simulink model "SalientPolePMSM"  (R2020b)
settings: Solver=VariableStepAuto  StartTime=0  StopTime=1  MaxStep=1e-4  RelTol=1e-4
values from neighbouring files (symbols this model uses):
  Bgain = 1    [DataSalientPolePMSM-DESKTOP-IINSHMA.m]    (also in DataSalientPolePMSM.m)
  Gcc_1ord = 1/(s/bandwidth(Gcc) + 1)    [DataSalientPolePMSM-DESKTOP-IINSHMA.m]    (also in DataSalientPolePMSM.m)
  lamdVec = mot.Ld*idVec+mot.lammg    [DataSalientPolePMSM-DESKTOP-IINSHMA.m]    (also in DataSalientPolePMSM.m)
  lamqVec = mot.Lq*iqVec    [DataSalientPolePMSM-DESKTOP-IINSHMA.m]    (also in DataSalientPolePMSM.m)
  TAB0_abc = Tabc_AB0^-1    [DataSalientPolePMSM-DESKTOP-IINSHMA.m]    (also in DataSalientPolePMSM.m)
  Tabc_AB0 = 2/3.*[     1       -1/2       -1/2 ... (first row only)    [DataSalientPolePMSM-DESKTOP-IINSHMA.m]    (also in DataSalientPolePMSM.m)
  Talphabeta_abc = Tabc_alphabeta^(-1)    [DataSalientPolePMSM-DESKTOP-IINSHMA.m]    (also in DataSalientPolePMSM.m)
undefined symbols (not defined in the file or in its folder): DiscIntNeverNeededParam, dqpll, inv, kid, kpd, magnitude, meas, mot, Obs, PI, stconv
libraries: simulink x53, pid_lib x3, powerlib x2, eeBldcCommutationLogic x1, electricdrivelib x1
(part 2 of 7)

== system SalientPolePMSM/DT SENSORLESS ALGORITHM DQ ==
  note: tangent PLL
  iabc1 : Inport
  udq_est : Inport  Port=2
  udq : Inport  Port=3
  In3 : Inport  Port=4
  thme1 : Inport  Port=5
  wme : Inport  Port=6
  Clarke + Park 5 : Subsystem
      settings: PortSchema="{\"entries\":[{\"content\":{\"sides\":[{\"content\":{\"connectorIds\":[\"In1\"]},\"type\":\"ConnectorPlacement.EquallySpacedRectSide\",\"uuid\":\"e456cd5a-7662-4e0b-a6c7-27ed01a0cde8\"},{\"content\":{\"connectorIds\":[\"Out1\"],\"side\":\"RIGHT\"},\"type\":\"ConnectorPlacement.EquallySpacedRectSide\",\"uuid\":\"028e266b-db3d-4fa0-9acb-55f4e679375c\"},{\"content\":{\"connectorIds\":[],\"side\":\"TOP\"},\"type\":\"ConnectorPlacement.EquallySpacedRectSide\",\"uuid\":\"fc8407b0-ab5c-4984-8f89-848ec890a8d5\"},{\"content\":{\"connectorIds\":[\"In2\"],\"side\":\"BOTTOM\"},\"type\":\"ConnectorPlacement.EquallySpacedRectSide\",\"uuid\":\"5b71beec-2170-4cb0-81b8-756f92b052d7\"},{\"content\":{\"connectorIds\":[],\"side\":\"HIDDEN\"},\"type\":\"ConnectorPlacement.EquallySpacedRectSide\",\"uuid\":\"110705d2-59f3-422e-b935-78b651f69ef1\"}]},\"type\":\"ConnectorPlacement.EquallySpacedConnector\",\"uuid\":\"4a76e66d-c848-4e9c-8e50-4d720647e920\"}],\"packageUris\":[\"http://schema.mathworks.com/mf0/Connector/R2020b\"],\"version\":\"1.0\"}"
  Classic PLL1 : Subsystem
  DECOUPLING : Subsystem
      settings: PortSchema="{\"entries\":[{\"content\":{\"sides\":[{\"content\":{\"connectorIds\":[\"In1\",\"In2\"]},\"type\":\"ConnectorPlacement.EquallySpacedRectSide\",\"uuid\":\"11caacf5-0bb5-4a8d-b3e9-7b1e88488e40\"},{\"content\":{\"connectorIds\":[\"Out1\",\"Out2\"],\"side\":\"RIGHT\"},\"type\":\"ConnectorPlacement.EquallySpacedRectSide\",\"uuid\":\"6263df69-80cd-4b04-a89b-dfca9161a93e\"},{\"content\":{\"connectorIds\":[],\"side\":\"TOP\"},\"type\":\"ConnectorPlacement.EquallySpacedRectSide\",\"uuid\":\"898c91db-8461-4171-8db9-87a99b66ce40\"},{\"content\":{\"connectorIds\":[\"In3\"],\"side\":\"BOTTOM\"},\"type\":\"ConnectorPlacement.EquallySpacedRectSide\",\"uuid\":\"185c1e28-6dbc-44e9-9bab-ce833de258e7\"},{\"content\":{\"connectorIds\":[],\"side\":\"HIDDEN\"},\"type\":\"ConnectorPlacement.EquallySpacedRectSide\",\"uuid\":\"0f2378b2-18e5-4bfa-bdaa-e448fe90a90d\"}]},\"type\":\"ConnectorPlacement.EquallySpacedConnector\",\"uuid\":\"5ac053f8-067e-460f-b603-fa451a6d3395\"}],\"packageUris\":[\"http://schema.mathworks.com/mf0/Connector/R2020b\"],\"version\":\"1.0\"}"
  Discrete Filter1 : DiscreteFilter  Numerator=[Obs.lpf.alpha*10]  Denominator=[1 ((Obs.lpf.alpha*10)-1)]  SampleTime=Obs.Ts
  Discrete Filter2 : DiscreteFilter  Commented=on  Numerator=[Obs.lpf.alpha]  Denominator=[1 (Obs.lpf.alpha-1)]  SampleTime=100e-6
  Discrete State-Space3 : DiscreteStateSpace  A=Obs.F1  B=Obs.G1  C=Obs.H1  D=Obs.D1  SampleTime=100e-6
  Discrete State-Space4 : DiscreteStateSpace  A=Obs.F1  B=Obs.G1  C=Obs.H1  D=Obs.D1  SampleTime=100e-6
  Discrete-Time Integrator : DiscreteIntegrator  gainval=1  SampleTime=100e-6  ICPrevOutput=DiscIntNeverNeededParam  ICPrevScaledInput=DiscIntNeverNeededParam
  Integrator : Integrator
  MATLAB Function1 : MATLAB Function  TreatAsAtomicUnit=on
  Normalized and improved PLL3 : Subsystem
  PII : Subsystem
      settings: PortSchema="{\"entries\":[{\"content\":{\"sides\":[{\"content\":{\"connectorIds\":[\"In1\"]},\"type\":\"ConnectorPlacement.EquallySpacedRectSide\",\"uuid\":\"b00016c6-1c57-43c7-9cfb-2a554e77d147\"},{\"content\":{\"connectorIds\":[\"Out1\"],\"side\":\"RIGHT\"},\"type\":\"ConnectorPlacement.EquallySpacedRectSide\",\"uuid\":\"2a623ad0-8b44-45a2-8fa5-d5134e76836f\"},{\"content\":{\"connectorIds\":[\"In2\"],\"side\":\"TOP\"},\"type\":\"ConnectorPlacement.EquallySpacedRectSide\",\"uuid\":\"30b77249-c9f6-4999-a309-d04d29204cea\"},{\"content\":{\"connectorIds\":[],\"side\":\"HIDDEN\"},\"type\":\"ConnectorPlacement.EquallySpacedRectSide\",\"uuid\":\"35f0e0cd-3c1e-4861-ab0d-8c8ad5904a85\"}]},\"type\":\"ConnectorPlacement.EquallySpacedConnector\",\"uuid\":\"0e7458ac-b887-4f57-92cf-b77cd1ee8214\"}],\"packageUris\":[\"http://schema.mathworks.com/mf0/Connector/R2020b\"],\"version\":\"1.0\"}"
  Rate Transition{,13..15} (4 alike) : RateTransition
  Rev_Park + Rev_Clarke1 : Subsystem
      settings: PortSchema="{\"entries\":[{\"content\":{\"sides\":[{\"content\":{\"connectorIds\":[\"In1\"]},\"type\":\"ConnectorPlacement.EquallySpacedRectSide\",\"uuid\":\"2aae3f04-c402-455e-9a5d-4c573bec95dc\"},{\"content\":{\"connectorIds\":[\"Out1\"],\"side\":\"RIGHT\"},\"type\":\"ConnectorPlacement.EquallySpacedRectSide\",\"uuid\":\"f1532c60-2267-456b-9c2f-34e60e60798d\"},{\"content\":{\"connectorIds\":[],\"side\":\"TOP\"},\"type\":\"ConnectorPlacement.EquallySpacedRectSide\",\"uuid\":\"04e1a6cc-513a-47f7-a63d-759add73a2e3\"},{\"content\":{\"connectorIds\":[\"In2\"],\"side\":\"BOTTOM\"},\"type\":\"ConnectorPlacement.EquallySpacedRectSide\",\"uuid\":\"e4fadd8d-bc98-4107-9436-b30fd69f2e4f\"},{\"content\":{\"connectorIds\":[],\"side\":\"HIDDEN\"},\"type\":\"ConnectorPlacement.EquallySpacedRectSide\",\"uuid\":\"086bd472-9627-4f82-bc83-4764e9943a88\"}]},\"type\":\"ConnectorPlacement.EquallySpacedConnector\",\"uuid\":\"0de85400-6c41-4ce8-8482-fdca09eb4650\"}],\"packageUris\":[\"http://schema.mathworks.com/mf0/Connector/R2020b\"],\"version\":\"1.0\"}"
  Scope : Scope  NumInputPorts=5
  Scope1 : Scope  NumInputPorts=3
  Scope2 : Scope
  Scope3 : Scope  NumInputPorts=3
  atan : MATLAB Function  TreatAsAtomicUnit=on
  thme_est : Outport
  wme_est : Outport  Port=2
  wires:
  Rate Transition14/1 -> Rev_Park + Rev_Clarke1/1(Iabc)
  Rate Transition15/1 -> Clarke + Park 5/1(abc)
  Rev_Park + Rev_Clarke1/1(dq) -> Scope2/1, DECOUPLING/1(idq_est)
  iabc1/1 -> Rate Transition14/1
  Rate Transition13/1 -> wme_est/1
  Discrete State-Space4/1 -> Classic PLL1/1(e_d), atan/1(ed), Scope/3
  Discrete State-Space3/1 -> Classic PLL1/2(e_q), atan/2(eq), Scope/4
  atan/1(thme) -> Scope3/3, PII/1(theta(k+1))
  DECOUPLING/1(ud' id) -> Scope/2, Discrete State-Space4/1
  DECOUPLING/2(uq' iq) -> Scope/1, Discrete State-Space3/1
  In3/1 -> Rate Transition15/1
  [THME_EST] -> Clarke + Park 5/2(thme)
  thme1/1 -> Scope3/1
  Discrete Filter1/1 -> Rate Transition13/1, DECOUPLING/3(wme_est)
  Rate Transition/1 -> thme_est/1
  Discrete-Time Integrator/1 -> Scope3/2, [THME_EST], Rate Transition/1
  PII/1(w_est) -> Discrete Filter1/1, Discrete-Time Integrator/1, MATLAB Function1/1(u)
  [THME_EST] -> Rev_Park + Rev_Clarke1/2(thme1)
  Clarke + Park 5/1(dq) -> DECOUPLING/2(udq_est)

== system SalientPolePMSM/Decoupling ==
  note: OUTPUT:
  note: INPUTS:
  udq* : Inport
  idq : Inport  Port=2
  wme : Inport  Port=3
  Demux : Demux  Outputs=2
  Demux1 : Demux  Outputs=2
  Demux2 : Demux  Outputs=2
  Gain : Gain  Gain=PI.cur.Ld
  Gain1 : Gain  Gain=PI.cur.Lq
  Gain2 : Gain  Gain=PI.cur.lammg
  Mux : Mux  Inputs=2
  Product : Product
  Product1 : Product
  Scope : Scope
  Scope1 : Scope
  Subtract : Sum  Inputs=-+
  Subtract1 : Sum  Inputs=+++
  Terminator1 : Terminator
  Terminator4 : Terminator
  idq1 : InportShadow  Port=2
  wme1 : InportShadow  Port=3
  udq** : Outport
  wires:
  Demux2/1 -> Product/2  "id"
  idq/1 -> Demux2/1
  Product/1 -> Subtract1/3  "wme*id*Ld"
  Subtract/1 -> Scope/1, Mux/1
  Demux/2 -> Subtract1/1
  Demux2/2 -> Terminator1/1
  Demux/1 -> Subtract/2
  wme/1 -> Gain/1, Gain2/1
  Subtract1/1 -> Scope1/1, Mux/2
  Gain2/1 -> Subtract1/2  "wme*lammg"
  Gain/1 -> Product/1
  Mux/1 -> udq**/1
  udq*/1 -> Demux/1
  Demux1/2 -> Product1/1  "iq"
  idq1/1 -> Demux1/1
  Demux1/1 -> Terminator4/1
  Gain1/1 -> Product1/2
  wme1/1 -> Gain1/1
  Product1/1 -> Subtract/1  "wme*iq*Lq"

== system SalientPolePMSM/Discrete SS ALGORITHM ==
  iabc : Inport
  uabc : Inport  Port=2
  ON_approx : Inport  Port=3
  ADD_integrator : Inport  Port=4
  DECOUPLING : Subsystem
      settings: PortSchema="{\"entries\":[{\"content\":{\"sides\":[{\"content\":{\"connectorIds\":[\"In1\",\"In2\"]},\"type\":\"ConnectorPlacement.EquallySpacedRectSide\",\"uuid\":\"11caacf5-0bb5-4a8d-b3e9-7b1e88488e40\"},{\"content\":{\"connectorIds\":[\"Out1\",\"Out2\"],\"side\":\"RIGHT\"},\"type\":\"ConnectorPlacement.EquallySpacedRectSide\",\"uuid\":\"6263df69-80cd-4b04-a89b-dfca9161a93e\"},{\"content\":{\"connectorIds\":[],\"side\":\"TOP\"},\"type\":\"ConnectorPlacement.EquallySpacedRectSide\",\"uuid\":\"898c91db-8461-4171-8db9-87a99b66ce40\"},{\"content\":{\"connectorIds\":[\"In3\"],\"side\":\"BOTTOM\"},\"type\":\"ConnectorPlacement.EquallySpacedRectSide\",\"uuid\":\"185c1e28-6dbc-44e9-9bab-ce833de258e7\"},{\"content\":{\"connectorIds\":[],\"side\":\"HIDDEN\"},\"type\":\"ConnectorPlacement.EquallySpacedRectSide\",\"uuid\":\"0f2378b2-18e5-4bfa-bdaa-e448fe90a90d\"}]},\"type\":\"ConnectorPlacement.EquallySpacedConnector\",\"uuid\":\"5ac053f8-067e-460f-b603-fa451a6d3395\"}],\"packageUris\":[\"http://schema.mathworks.com/mf0/Connector/R2020b\"],\"version\":\"1.0\"}"
  Demux : Demux  Outputs=2
  Discrete Filter2 : DiscreteFilter  Numerator=[dqpll.lpf.alpha]  Denominator=[1 (dqpll.lpf.alpha-1)]
  Discrete State-Space1 : DiscreteStateSpace  A=dqpll.est.F1  B=dqpll.est.G1  C=dqpll.est.H1  D=dqpll.est.D1  SampleTime=dqpll.Ts
  Discrete State-Space2 : DiscreteStateSpace  A=dqpll.est.F1  B=dqpll.est.G1  C=dqpll.est.H1  D=dqpll.est.D1  SampleTime=dqpll.Ts
  Discrete-Time Integrator1 : DiscreteIntegrator  gainval=1  SampleTime=dqpll.Ts  ICPrevOutput=DiscIntNeverNeededParam  ICPrevScaledInput=DiscIntNeverNeededParam
  MATLAB Function3 : MATLAB Function  TreatAsAtomicUnit=on
  PI : Subsystem
  PII : Subsystem
  Rate Transition{,1..5} (6 alike) : RateTransition
  Scope : Scope  NumInputPorts=2
  Scope1 : Scope  NumInputPorts=2
  Subsystem5 : Subsystem
      settings: PortSchema="{\"entries\":[{\"content\":{\"sides\":[{\"content\":{\"connectorIds\":[\"In1\"]},\"type\":\"ConnectorPlacement.EquallySpacedRectSide\",\"uuid\":\"4ed90ab9-1fa1-426e-9a51-633f86eaed93\"},{\"content\":{\"connectorIds\":[\"Out1\"],\"side\":\"RIGHT\"},\"type\":\"ConnectorPlacement.EquallySpacedRectSide\",\"uuid\":\"a783641a-eefd-4804-96bc-e093b09f1b23\"},{\"content\":{\"connectorIds\":[\"In2\"],\"side\":\"TOP\"},\"type\":\"ConnectorPlacement.EquallySpacedRectSide\",\"uuid\":\"b71fad55-6d7c-4fa9-b8c9-7c2d781b5980\"},{\"content\":{\"connectorIds\":[],\"side\":\"BOTTOM\"},\"type\":\"ConnectorPlacement.EquallySpacedRectSide\",\"uuid\":\"0ef0ee48-37c5-4f1f-a4a0-75388778f62a\"},{\"content\":{\"connectorIds\":[],\"side\":\"HIDDEN\"},\"type\":\"ConnectorPlacement.EquallySpacedRectSide\",\"uuid\":\"d9128c0c-5cc0-40ee-9c52-e819b4b0207f\"}]},\"type\":\"ConnectorPlacement.EquallySpacedConnector\",\"uuid\":\"84170b20-7cd7-4bfe-ad20-891cbad09232\"}],\"packageUris\":[\"http://schema.mathworks.com/mf0/Connector/R2020b\"],\"version\":\"1.0\"}"
  Subsystem6 : Subsystem
      settings: PortSchema="{\"entries\":[{\"content\":{\"sides\":[{\"content\":{\"connectorIds\":[\"In1\"]},\"type\":\"ConnectorPlacement.EquallySpacedRectSide\",\"uuid\":\"4ed90ab9-1fa1-426e-9a51-633f86eaed93\"},{\"content\":{\"connectorIds\":[\"Out1\"],\"side\":\"RIGHT\"},\"type\":\"ConnectorPlacement.EquallySpacedRectSide\",\"uuid\":\"a783641a-eefd-4804-96bc-e093b09f1b23\"},{\"content\":{\"connectorIds\":[],\"side\":\"TOP\"},\"type\":\"ConnectorPlacement.EquallySpacedRectSide\",\"uuid\":\"b71fad55-6d7c-4fa9-b8c9-7c2d781b5980\"},{\"content\":{\"connectorIds\":[\"In2\"],\"side\":\"BOTTOM\"},\"type\":\"ConnectorPlacement.EquallySpacedRectSide\",\"uuid\":\"0ef0ee48-37c5-4f1f-a4a0-75388778f62a\"},{\"content\":{\"connectorIds\":[],\"side\":\"HIDDEN\"},\"type\":\"ConnectorPlacement.EquallySpacedRectSide\",\"uuid\":\"d9128c0c-5cc0-40ee-9c52-e819b4b0207f\"}]},\"type\":\"ConnectorPlacement.EquallySpacedConnector\",\"uuid\":\"84170b20-7cd7-4bfe-ad20-891cbad09232\"}],\"packageUris\":[\"http://schema.mathworks.com/mf0/Connector/R2020b\"],\"version\":\"1.0\"}"
  Switch : Switch  Criteria=u2 > Threshold
  Switch1 : Switch  Criteria=u2 > Threshold
  Terminator : Terminator
  atan : MATLAB Function  TreatAsAtomicUnit=on
  atanApprox : MATLAB Function  TreatAsAtomicUnit=on
  thme_est : Outport
  wme_est : Outport  Port=2
  wires:
  Discrete-Time Integrator1/1 -> [THME_EST], Rate Transition/1
  uabc/1 -> Rate Transition3/1
  iabc/1 -> Rate Transition2/1
  Rate Transition/1 -> thme_est/1
  Rate Transition1/1 -> wme_est/1
  Rate Transition2/1 -> Subsystem5/1(abc)
  Rate Transition3/1 -> Subsystem6/1(abc)
  Discrete Filter2/1 -> Rate Transition1/1, DECOUPLING/3(wme_est), atanApprox/3(wme_est)
  Switch1/1 -> MATLAB Function3/1(u)
  Discrete State-Space2/1 -> atanApprox/2(ed), Scope/2, atan/1(ed)
  atan/1(thme) -> Switch/3
  Discrete State-Space1/1 -> Scope/1, atan/2(eq)
  Subsystem5/1(dq) -> Demux/1, Scope1/2, DECOUPLING/1(idq_est)
  Subsystem6/1(dq) -> Scope1/1, DECOUPLING/2(udq_est)
  DECOUPLING/1(ud' id) -> Discrete State-Space2/1
  DECOUPLING/2(uq' iq) -> Discrete State-Space1/1
  [THME_EST] -> Subsystem5/2(thme), Subsystem6/2(thme)
  atanApprox/1(thme) -> Switch/1
  ON_approx/1 -> Rate Transition4/1
  Demux/2 -> Terminator/1
  Demux/1 -> atanApprox/1(id)
  Rate Transition4/1 -> Switch/2
  PII/1(w_est) -> Switch1/1
  PI/1(w_est) -> Switch1/3
  ADD_integrator/1 -> Rate Transition5/1
  Switch/1 -> PII/1(e), PI/1(e)
  Rate Transition5/1 -> Switch1/2
  MATLAB Function3/1(y) -> Discrete-Time Integrator1/1, Discrete Filter2/1

== system SalientPolePMSM/Discrete SS ALGORITHM1 ==
  iabc : Inport
  uabc : Inport  Port=2
  ON_approx : Inport  Port=3
  ADD_integrator : Inport  Port=4
  DECOUPLING : Subsystem
      settings: PortSchema="{\"entries\":[{\"content\":{\"sides\":[{\"content\":{\"connectorIds\":[\"In1\",\"In2\"]},\"type\":\"ConnectorPlacement.EquallySpacedRectSide\",\"uuid\":\"11caacf5-0bb5-4a8d-b3e9-7b1e88488e40\"},{\"content\":{\"connectorIds\":[\"Out1\",\"Out2\"],\"side\":\"RIGHT\"},\"type\":\"ConnectorPlacement.EquallySpacedRectSide\",\"uuid\":\"6263df69-80cd-4b04-a89b-dfca9161a93e\"},{\"content\":{\"connectorIds\":[],\"side\":\"TOP\"},\"type\":\"ConnectorPlacement.EquallySpacedRectSide\",\"uuid\":\"898c91db-8461-4171-8db9-87a99b66ce40\"},{\"content\":{\"connectorIds\":[\"In3\"],\"side\":\"BOTTOM\"},\"type\":\"ConnectorPlacement.EquallySpacedRectSide\",\"uuid\":\"185c1e28-6dbc-44e9-9bab-ce833de258e7\"},{\"content\":{\"connectorIds\":[],\"side\":\"HIDDEN\"},\"type\":\"ConnectorPlacement.EquallySpacedRectSide\",\"uuid\":\"0f2378b2-18e5-4bfa-bdaa-e448fe90a90d\"}]},\"type\":\"ConnectorPlacement.EquallySpacedConnector\",\"uuid\":\"5ac053f8-067e-460f-b603-fa451a6d3395\"}],\"packageUris\":[\"http://schema.mathworks.com/mf0/Connector/R2020b\"],\"version\":\"1.0\"}"
  Demux : Demux  Outputs=2
  Discrete Filter2 : DiscreteFilter  Numerator=[dqpll.lpf.alpha]  Denominator=[1 (dqpll.lpf.alpha-1)]
  Discrete State-Space1 : DiscreteStateSpace  A=dqpll.est.F1  B=dqpll.est.G1  C=dqpll.est.H1  D=dqpll.est.D1  SampleTime=dqpll.Ts
  Discrete State-Space2 : DiscreteStateSpace  A=dqpll.est.F1  B=dqpll.est.G1  C=dqpll.est.H1  D=dqpll.est.D1  SampleTime=dqpll.Ts
  Discrete-Time Integrator1 : DiscreteIntegrator  gainval=1  SampleTime=dqpll.Ts  ICPrevOutput=DiscIntNeverNeededParam  ICPrevScaledInput=DiscIntNeverNeededParam
  PI : Subsystem
  PII : Subsystem
  Rate Transition{,1..5} (6 alike) : RateTransition
  Subsystem5 : Subsystem
      settings: PortSchema="{\"entries\":[{\"content\":{\"sides\":[{\"content\":{\"connectorIds\":[\"In1\"]},\"type\":\"ConnectorPlacement.EquallySpacedRectSide\",\"uuid\":\"4ed90ab9-1fa1-426e-9a51-633f86eaed93\"},{\"content\":{\"connectorIds\":[\"Out1\"],\"side\":\"RIGHT\"},\"type\":\"ConnectorPlacement.EquallySpacedRectSide\",\"uuid\":\"a783641a-eefd-4804-96bc-e093b09f1b23\"},{\"content\":{\"connectorIds\":[\"In2\"],\"side\":\"TOP\"},\"type\":\"ConnectorPlacement.EquallySpacedRectSide\",\"uuid\":\"b71fad55-6d7c-4fa9-b8c9-7c2d781b5980\"},{\"content\":{\"connectorIds\":[],\"side\":\"BOTTOM\"},\"type\":\"ConnectorPlacement.EquallySpacedRectSide\",\"uuid\":\"0ef0ee48-37c5-4f1f-a4a0-75388778f62a\"},{\"content\":{\"connectorIds\":[],\"side\":\"HIDDEN\"},\"type\":\"ConnectorPlacement.EquallySpacedRectSide\",\"uuid\":\"d9128c0c-5cc0-40ee-9c52-e819b4b0207f\"}]},\"type\":\"ConnectorPlacement.EquallySpacedConnector\",\"uuid\":\"84170b20-7cd7-4bfe-ad20-891cbad09232\"}],\"packageUris\":[\"http://schema.mathworks.com/mf0/Connector/R2020b\"],\"version\":\"1.0\"}"
  Subsystem6 : Subsystem
      settings: PortSchema="{\"entries\":[{\"content\":{\"sides\":[{\"content\":{\"connectorIds\":[\"In1\"]},\"type\":\"ConnectorPlacement.EquallySpacedRectSide\",\"uuid\":\"4ed90ab9-1fa1-426e-9a51-633f86eaed93\"},{\"content\":{\"connectorIds\":[\"Out1\"],\"side\":\"RIGHT\"},\"type\":\"ConnectorPlacement.EquallySpacedRectSide\",\"uuid\":\"a783641a-eefd-4804-96bc-e093b09f1b23\"},{\"content\":{\"connectorIds\":[],\"side\":\"TOP\"},\"type\":\"ConnectorPlacement.EquallySpacedRectSide\",\"uuid\":\"b71fad55-6d7c-4fa9-b8c9-7c2d781b5980\"},{\"content\":{\"connectorIds\":[\"In2\"],\"side\":\"BOTTOM\"},\"type\":\"ConnectorPlacement.EquallySpacedRectSide\",\"uuid\":\"0ef0ee48-37c5-4f1f-a4a0-75388778f62a\"},{\"content\":{\"connectorIds\":[],\"side\":\"HIDDEN\"},\"type\":\"ConnectorPlacement.EquallySpacedRectSide\",\"uuid\":\"d9128c0c-5cc0-40ee-9c52-e819b4b0207f\"}]},\"type\":\"ConnectorPlacement.EquallySpacedConnector\",\"uuid\":\"84170b20-7cd7-4bfe-ad20-891cbad09232\"}],\"packageUris\":[\"http://schema.mathworks.com/mf0/Connector/R2020b\"],\"version\":\"1.0\"}"
  Switch : Switch  Criteria=u2 > Threshold
  Switch1 : Switch  Criteria=u2 > Threshold
  Terminator : Terminator
  atan : MATLAB Function  TreatAsAtomicUnit=on
  atanApprox : MATLAB Function  TreatAsAtomicUnit=on
  thme_est : Outport
  wme_est : Outport  Port=2
  wires:
  Discrete-Time Integrator1/1 -> [THME_EST], Rate Transition/1
  uabc/1 -> Rate Transition3/1
  iabc/1 -> Rate Transition2/1
  Rate Transition/1 -> thme_est/1
  Rate Transition1/1 -> wme_est/1
  Rate Transition2/1 -> Subsystem5/1(abc)
  Rate Transition3/1 -> Subsystem6/1(abc)
  Discrete Filter2/1 -> Rate Transition1/1, DECOUPLING/3(wme_est), atanApprox/3(wme_est)
  Switch1/1 -> Discrete-Time Integrator1/1, Discrete Filter2/1
  Discrete State-Space2/1 -> atanApprox/2(ed), atan/1(ed)
  atan/1(thme) -> Switch/3
  Discrete State-Space1/1 -> atan/2(eq)
  Subsystem5/1(dq) -> Demux/1, DECOUPLING/1(idq_est)
  Subsystem6/1(dq) -> DECOUPLING/2(udq_est)
  DECOUPLING/1(ud' id) -> Discrete State-Space2/1
  DECOUPLING/2(uq' iq) -> Discrete State-Space1/1
  [THME_EST] -> Subsystem5/2(thme), Subsystem6/2(thme)
  atanApprox/1(thme) -> Switch/1
  ON_approx/1 -> Rate Transition4/1
  Demux/2 -> Terminator/1
  Demux/1 -> atanApprox/1(id)
  Rate Transition4/1 -> Switch/2
  PII/1(w_est) -> Switch1/1
  PI/1(w_est) -> Switch1/3
  ADD_integrator/1 -> Rate Transition5/1
  Switch/1 -> PII/1(e), PI/1(e)
  Rate Transition5/1 -> Switch1/2

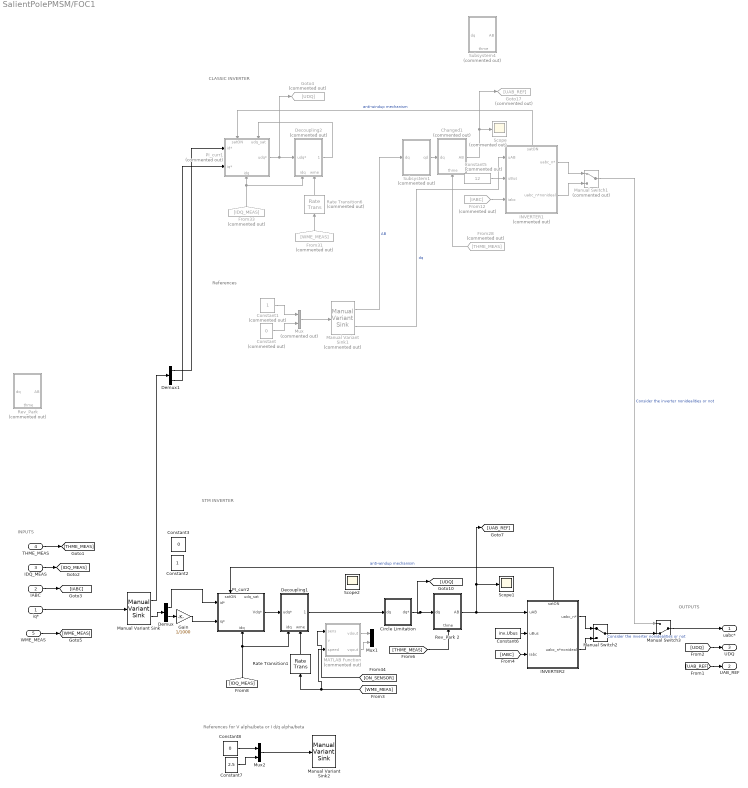
== system SalientPolePMSM/FOC1 ==
  note: References for V alpha/beta or I d/q alpha/beta
  note: OUTPUTS
  note: STM INVERTER
  note: INPUTS
  note: CLASSIC INVERTER
  note: References
  iq* : Inport
  IABC : Inport  Port=2
  IDQ_MEAS : Inport  Port=3
  THME_MEAS : Inport  Port=4
  WME_MEAS : Inport  Port=5
  Changed1 : Subsystem  Commented=on
      settings: PortSchema="{\"entries\":[{\"content\":{\"sides\":[{\"content\":{\"connectorIds\":[\"In1\"]},\"type\":\"ConnectorPlacement.EquallySpacedRectSide\",\"uuid\":\"ea71606c-027e-481e-aba4-13f62585a677\"},{\"content\":{\"connectorIds\":[\"Out1\"],\"side\":\"RIGHT\"},\"type\":\"ConnectorPlacement.EquallySpacedRectSide\",\"uuid\":\"049929a5-aa1b-4856-95c9-17d9e38685d8\"},{\"content\":{\"connectorIds\":[],\"side\":\"TOP\"},\"type\":\"ConnectorPlacement.EquallySpacedRectSide\",\"uuid\":\"6c7bede6-8f52-43d3-8925-2a8f1f9ce837\"},{\"content\":{\"connectorIds\":[\"In2\"],\"side\":\"BOTTOM\"},\"type\":\"ConnectorPlacement.EquallySpacedRectSide\",\"uuid\":\"34422c14-5aba-4255-be55-6ec9502f5391\"},{\"content\":{\"connectorIds\":[],\"side\":\"HIDDEN\"},\"type\":\"ConnectorPlacement.EquallySpacedRectSide\",\"uuid\":\"23931446-a8a1-432e-a504-22fe56898a45\"}]},\"type\":\"ConnectorPlacement.EquallySpacedConnector\",\"uuid\":\"f447a990-15af-42ca-9219-73ae62b099f5\"}],\"packageUris\":[\"http://schema.mathworks.com/mf0/Connector/R2020b\"],\"version\":\"1.0\"}"
  Circle Limitation : Subsystem
  Constant : Constant  Commented=on  Value=0  SampleTime=inv.Ts
  Constant1 : Constant  Commented=on  SampleTime=inv.Ts
  Constant2 : Constant  SampleTime=-1
  Constant3 : Constant  Value=0  SampleTime=-1
  Constant5 : Constant  Commented=on  Value=12
  Constant6 : Constant  Value=inv.Ubus
  Constant7 : Constant  Value=2.5  SampleTime=-1
  Constant8 : Constant  Value=0  SampleTime=-1
  Decoupling1 : Subsystem
      settings: PortSchema="{\"entries\":[{\"content\":{\"sides\":[{\"content\":{\"connectorIds\":[\"In1\"]},\"type\":\"ConnectorPlacement.EquallySpacedRectSide\",\"uuid\":\"366d4760-99ea-4839-93ce-cd028ffff2ed\"},{\"content\":{\"connectorIds\":[\"Out1\"],\"side\":\"RIGHT\"},\"type\":\"ConnectorPlacement.EquallySpacedRectSide\",\"uuid\":\"ffb80cd0-5569-4ccd-9b8e-dc37fbe2d6f7\"},{\"content\":{\"connectorIds\":[],\"side\":\"TOP\"},\"type\":\"ConnectorPlacement.EquallySpacedRectSide\",\"uuid\":\"2e02478e-0c74-4c41-9c3e-8c0e6bb6923b\"},{\"content\":{\"connectorIds\":[\"In2\",\"In3\"],\"side\":\"BOTTOM\"},\"type\":\"ConnectorPlacement.EquallySpacedRectSide\",\"uuid\":\"0c356034-c9d0-432b-942d-38470146113e\"}]},\"type\":\"ConnectorPlacement.EquallySpacedConnector\",\"uuid\":\"999d36d2-be3d-4c0f-9dc8-4c30e8aa3320\"}],\"packageUris\":[\"http://schema.mathworks.com/mf0/Connector/19700101\"],\"version\":\"1.0\"}"
  Decoupling2 : Subsystem  Commented=on
      settings: PortSchema="{\"entries\":[{\"content\":{\"sides\":[{\"content\":{\"connectorIds\":[\"In1\"]},\"type\":\"ConnectorPlacement.EquallySpacedRectSide\",\"uuid\":\"366d4760-99ea-4839-93ce-cd028ffff2ed\"},{\"content\":{\"connectorIds\":[\"Out1\"],\"side\":\"RIGHT\"},\"type\":\"ConnectorPlacement.EquallySpacedRectSide\",\"uuid\":\"ffb80cd0-5569-4ccd-9b8e-dc37fbe2d6f7\"},{\"content\":{\"connectorIds\":[],\"side\":\"TOP\"},\"type\":\"ConnectorPlacement.EquallySpacedRectSide\",\"uuid\":\"2e02478e-0c74-4c41-9c3e-8c0e6bb6923b\"},{\"content\":{\"connectorIds\":[\"In2\",\"In3\"],\"side\":\"BOTTOM\"},\"type\":\"ConnectorPlacement.EquallySpacedRectSide\",\"uuid\":\"0c356034-c9d0-432b-942d-38470146113e\"}]},\"type\":\"ConnectorPlacement.EquallySpacedConnector\",\"uuid\":\"999d36d2-be3d-4c0f-9dc8-4c30e8aa3320\"}],\"packageUris\":[\"http://schema.mathworks.com/mf0/Connector/19700101\"],\"version\":\"1.0\"}"
  Demux : Demux  Outputs=2
  Demux1 : Demux  Outputs=2
  From12 : From  Commented=on  GotoTag=IABC
  From28 : From  Commented=on  GotoTag=THME_MEAS
  From31 : From  Commented=on  GotoTag=WME_MEAS
  From33 : From  Commented=on  GotoTag=IDQ_MEAS
  Gain : Gain  Gain=1/1000
  Goto17 : Goto  Commented=on  GotoTag=UAB_REF
  Goto4 : Goto  Commented=on  GotoTag=UDQ
  INVERTER1 : Subsystem  Commented=on
      settings: PortSchema="{\"entries\":[{\"content\":{\"sides\":[{\"content\":{\"connectorIds\":[\"In1\",\"In2\",\"In3\"]},\"type\":\"ConnectorPlacement.EquallySpacedRectSide\",\"uuid\":\"79c77d12-022f-42ce-98d0-f3ead9d04a95\"},{\"content\":{\"connectorIds\":[\"Out1\",\"Out2\"],\"side\":\"RIGHT\"},\"type\":\"ConnectorPlacement.EquallySpacedRectSide\",\"uuid\":\"afd498dc-a72a-45ee-96a4-44488bf591ce\"},{\"content\":{\"connectorIds\":[\"Out3\"],\"side\":\"TOP\"},\"type\":\"ConnectorPlacement.EquallySpacedRectSide\",\"uuid\":\"f8f8ad46-d0da-4286-941c-855cc15ed51d\"}]},\"type\":\"ConnectorPlacement.EquallySpacedConnector\",\"uuid\":\"436ef73d-4718-409e-82fb-57ff2ccd93cf\"}],\"packageUris\":[\"http://schema.mathworks.com/mf0/Connector/R2020b\"],\"version\":\"1.0\"}"
  INVERTER2 : Subsystem
      settings: PortSchema="{\"entries\":[{\"content\":{\"sides\":[{\"content\":{\"connectorIds\":[\"In1\",\"In2\",\"In3\"]},\"type\":\"ConnectorPlacement.EquallySpacedRectSide\",\"uuid\":\"79c77d12-022f-42ce-98d0-f3ead9d04a95\"},{\"content\":{\"connectorIds\":[\"Out1\",\"Out2\"],\"side\":\"RIGHT\"},\"type\":\"ConnectorPlacement.EquallySpacedRectSide\",\"uuid\":\"afd498dc-a72a-45ee-96a4-44488bf591ce\"},{\"content\":{\"connectorIds\":[\"Out3\"],\"side\":\"TOP\"},\"type\":\"ConnectorPlacement.EquallySpacedRectSide\",\"uuid\":\"f8f8ad46-d0da-4286-941c-855cc15ed51d\"}]},\"type\":\"ConnectorPlacement.EquallySpacedConnector\",\"uuid\":\"436ef73d-4718-409e-82fb-57ff2ccd93cf\"}],\"packageUris\":[\"http://schema.mathworks.com/mf0/Connector/R2020b\"],\"version\":\"1.0\"}"
  MATLAB Function : MATLAB Function  Commented=on  TreatAsAtomicUnit=on  SystemSampleTime=inv.Ts
  Manual Variant Sink : simulink/Signal Routing/Manual Variant Sink  NumChoices=2  LabelModeActiveChoice=V_2
  Manual Variant Sink1 : simulink/Signal Routing/Manual Variant Sink  Commented=on  NumChoices=2  LabelModeActiveChoice=V_2
  Manual Variant Sink2 : simulink/Signal Routing/Manual Variant Sink  NumChoices=2  LabelModeActiveChoice=V_1
  Manual Switch1 : ManualSwitch  Commented=on
  Manual Switch2 : ManualSwitch
  Manual Switch3 : ManualSwitch  CurrentSetting=0
  Mux : Mux  Commented=on  Inputs=2
  Mux1 : Mux  Inputs=2
  Mux2 : Mux  Inputs=2
  PI_curr1 : Subsystem  Commented=on
      settings: PortSchema="{\"entries\":[{\"content\":{\"sides\":[{\"content\":{\"connectorIds\":[\"In1\",\"In2\"]},\"type\":\"ConnectorPlacement.EquallySpacedRectSide\",\"uuid\":\"366d4760-99ea-4839-93ce-cd028ffff2ed\"},{\"content\":{\"connectorIds\":[\"Out1\"],\"side\":\"RIGHT\"},\"type\":\"ConnectorPlacement.EquallySpacedRectSide\",\"uuid\":\"ffb80cd0-5569-4ccd-9b8e-dc37fbe2d6f7\"},{\"content\":{\"connectorIds\":[\"In3\",\"In4\"],\"side\":\"TOP\"},\"type\":\"ConnectorPlacement.EquallySpacedRectSide\",\"uuid\":\"2e02478e-0c74-4c41-9c3e-8c0e6bb6923b\"},{\"content\":{\"connectorIds\":[\"In5\"],\"side\":\"BOTTOM\"},\"type\":\"ConnectorPlacement.EquallySpacedRectSide\",\"uuid\":\"f2f25d95-a140-4291-ad57-573bdd6b43a2\"}]},\"type\":\"ConnectorPlacement.EquallySpacedConnector\",\"uuid\":\"999d36d2-be3d-4c0f-9dc8-4c30e8aa3320\"}],\"packageUris\":[\"http://schema.mathworks.com/mf0/Connector/R2020b\"],\"version\":\"1.0\"}"
  PI_curr2 : Subsystem
      settings: PortSchema="{\"entries\":[{\"content\":{\"sides\":[{\"content\":{\"connectorIds\":[\"In1\",\"In2\"]},\"type\":\"ConnectorPlacement.EquallySpacedRectSide\",\"uuid\":\"366d4760-99ea-4839-93ce-cd028ffff2ed\"},{\"content\":{\"connectorIds\":[\"Out1\"],\"side\":\"RIGHT\"},\"type\":\"ConnectorPlacement.EquallySpacedRectSide\",\"uuid\":\"ffb80cd0-5569-4ccd-9b8e-dc37fbe2d6f7\"},{\"content\":{\"connectorIds\":[\"In3\",\"In4\"],\"side\":\"TOP\"},\"type\":\"ConnectorPlacement.EquallySpacedRectSide\",\"uuid\":\"2e02478e-0c74-4c41-9c3e-8c0e6bb6923b\"},{\"content\":{\"connectorIds\":[\"In5\"],\"side\":\"BOTTOM\"},\"type\":\"ConnectorPlacement.EquallySpacedRectSide\",\"uuid\":\"f2f25d95-a140-4291-ad57-573bdd6b43a2\"}]},\"type\":\"ConnectorPlacement.EquallySpacedConnector\",\"uuid\":\"999d36d2-be3d-4c0f-9dc8-4c30e8aa3320\"}],\"packageUris\":[\"http://schema.mathworks.com/mf0/Connector/R2020b\"],\"version\":\"1.0\"}"
  Rate Transition1 : RateTransition  OutPortSampleTime=PI.cur.Ts
  Rate Transition6 : RateTransition  Commented=on  OutPortSampleTime=PI.cur.Ts
  Rev_Park : Subsystem  Commented=on
      settings: PortSchema="{\"entries\":[{\"content\":{\"sides\":[{\"content\":{\"connectorIds\":[\"In1\"]},\"type\":\"ConnectorPlacement.EquallySpacedRectSide\",\"uuid\":\"ea71606c-027e-481e-aba4-13f62585a677\"},{\"content\":{\"connectorIds\":[\"Out1\"],\"side\":\"RIGHT\"},\"type\":\"ConnectorPlacement.EquallySpacedRectSide\",\"uuid\":\"049929a5-aa1b-4856-95c9-17d9e38685d8\"},{\"content\":{\"connectorIds\":[],\"side\":\"TOP\"},\"type\":\"ConnectorPlacement.EquallySpacedRectSide\",\"uuid\":\"6c7bede6-8f52-43d3-8925-2a8f1f9ce837\"},{\"content\":{\"connectorIds\":[\"In2\"],\"side\":\"BOTTOM\"},\"type\":\"ConnectorPlacement.EquallySpacedRectSide\",\"uuid\":\"34422c14-5aba-4255-be55-6ec9502f5391\"},{\"content\":{\"connectorIds\":[],\"side\":\"HIDDEN\"},\"type\":\"ConnectorPlacement.EquallySpacedRectSide\",\"uuid\":\"23931446-a8a1-432e-a504-22fe56898a45\"}]},\"type\":\"ConnectorPlacement.EquallySpacedConnector\",\"uuid\":\"f447a990-15af-42ca-9219-73ae62b099f5\"}],\"packageUris\":[\"http://schema.mathworks.com/mf0/Connector/R2020b\"],\"version\":\"1.0\"}"
  Rev_Park 2 : Subsystem
      settings: PortSchema="{\"entries\":[{\"content\":{\"sides\":[{\"content\":{\"connectorIds\":[\"In1\"]},\"type\":\"ConnectorPlacement.EquallySpacedRectSide\",\"uuid\":\"ea71606c-027e-481e-aba4-13f62585a677\"},{\"content\":{\"connectorIds\":[\"Out1\"],\"side\":\"RIGHT\"},\"type\":\"ConnectorPlacement.EquallySpacedRectSide\",\"uuid\":\"049929a5-aa1b-4856-95c9-17d9e38685d8\"},{\"content\":{\"connectorIds\":[],\"side\":\"TOP\"},\"type\":\"ConnectorPlacement.EquallySpacedRectSide\",\"uuid\":\"6c7bede6-8f52-43d3-8925-2a8f1f9ce837\"},{\"content\":{\"connectorIds\":[\"In2\"],\"side\":\"BOTTOM\"},\"type\":\"ConnectorPlacement.EquallySpacedRectSide\",\"uuid\":\"34422c14-5aba-4255-be55-6ec9502f5391\"},{\"content\":{\"connectorIds\":[],\"side\":\"HIDDEN\"},\"type\":\"ConnectorPlacement.EquallySpacedRectSide\",\"uuid\":\"23931446-a8a1-432e-a504-22fe56898a45\"}]},\"type\":\"ConnectorPlacement.EquallySpacedConnector\",\"uuid\":\"f447a990-15af-42ca-9219-73ae62b099f5\"}],\"packageUris\":[\"http://schema.mathworks.com/mf0/Connector/R2020b\"],\"version\":\"1.0\"}"
  Scope : Scope  Commented=on
  Scope1 : Scope
  Scope2 : Scope
  Subsystem1 : Subsystem  Commented=on
  Subsystem4 : Subsystem  Commented=on
      settings: PortSchema="{\"entries\":[{\"content\":{\"sides\":[{\"content\":{\"connectorIds\":[\"In1\"]},\"type\":\"ConnectorPlacement.EquallySpacedRectSide\",\"uuid\":\"ea71606c-027e-481e-aba4-13f62585a677\"},{\"content\":{\"connectorIds\":[\"Out1\"],\"side\":\"RIGHT\"},\"type\":\"ConnectorPlacement.EquallySpacedRectSide\",\"uuid\":\"049929a5-aa1b-4856-95c9-17d9e38685d8\"},{\"content\":{\"connectorIds\":[],\"side\":\"TOP\"},\"type\":\"ConnectorPlacement.EquallySpacedRectSide\",\"uuid\":\"6c7bede6-8f52-43d3-8925-2a8f1f9ce837\"},{\"content\":{\"connectorIds\":[\"In2\"],\"side\":\"BOTTOM\"},\"type\":\"ConnectorPlacement.EquallySpacedRectSide\",\"uuid\":\"34422c14-5aba-4255-be55-6ec9502f5391\"},{\"content\":{\"connectorIds\":[],\"side\":\"HIDDEN\"},\"type\":\"ConnectorPlacement.EquallySpacedRectSide\",\"uuid\":\"23931446-a8a1-432e-a504-22fe56898a45\"}]},\"type\":\"ConnectorPlacement.EquallySpacedConnector\",\"uuid\":\"f447a990-15af-42ca-9219-73ae62b099f5\"}],\"packageUris\":[\"http://schema.mathworks.com/mf0/Connector/R2020b\"],\"version\":\"1.0\"}"
  uabc* : Outport
  UAB_REF : Outport  Port=2
  UDQ : Outport  Port=3
  wires:
  Constant6/1 -> INVERTER2/2(uBus)
  INVERTER2/3(satON) -> PI_curr2/3(satON)  "anti-windup mechanism"
  INVERTER2/1(uabc_n*) -> Manual Switch2/1
  INVERTER2/2(uabc_n*nonideal) -> Manual Switch2/2
  [IABC] -> INVERTER2/3(iabc)
  [IDQ_MEAS] -> Decoupling1/2(idq), PI_curr2/5(idq)
  Constant/1 -> Mux/2
  Constant1/1 -> Mux/1
  Demux1/1 -> PI_curr1/1(id*)
  [UDQ] -> UDQ/1
  THME_MEAS/1 -> [THME_MEAS]
  IDQ_MEAS/1 -> [IDQ_MEAS]
  IABC/1 -> [IABC]
  [UAB_REF] -> UAB_REF/1
  Decoupling2/1(udq**) -> PI_curr1/4(udq_sat)
  Rate Transition6/1 -> Decoupling2/3(wme)
  Constant5/1 -> INVERTER1/2(uBus)
  INVERTER1/1(uabc_n*) -> Manual Switch1/1
  From28/1 -> Changed1/2(thme)
  INVERTER1/2(uabc_n*nonideal) -> Manual Switch1/2
  INVERTER1/3(satON) -> PI_curr1/3(satON)  "anti-windup mechanism"
  Changed1/1(AB) -> Scope/1, Goto17/1
  From31/1 -> Rate Transition6/1
  From33/1 -> Decoupling2/2(idq), PI_curr1/5(idq)
  From12/1 -> INVERTER1/3(iabc)
  PI_curr1/1(udq*) -> Decoupling2/1(udq*), Goto4/1
  Subsystem1/1(qd) -> Changed1/1(dq)
  [WME_MEAS] -> MATLAB Function/3(speed), Rate Transition1/1
  Manual Switch3/1 -> uabc*/1
  Manual Switch2/1 -> Manual Switch3/2  "Consider the inverter nonidealities or not"
  Manual Switch1/1 -> Manual Switch3/1  "Consider the inverter nonidealities or not"
  iq*/1 -> Manual Variant Sink/1
  Mux/1 -> Manual Variant Sink1/1
  Manual Variant Sink1/1 -> Subsystem1/1(dq)  "AB"
  Manual Variant Sink1/2 -> INVERTER1/1(uAB)  "dq"
  Mux2/1 -> Manual Variant Sink2/1
  Rev_Park 2/1(AB) -> INVERTER2/1(uAB), [UAB_REF], Scope1/1
  Manual Variant Sink/2 -> Demux/1
  Manual Variant Sink/1 -> Demux1/1
  Demux1/2 -> PI_curr1/2(iq*)
  WME_MEAS/1 -> [WME_MEAS]
  [THME_MEAS] -> Rev_Park 2/2(thme)
  [ON_SENSOR] -> MATLAB Function/1(sens)
  MATLAB Function/2(vqout) -> Mux1/2
  MATLAB Function/1(vdout) -> Mux1/1
  Constant7/1 -> Mux2/2
  Constant8/1 -> Mux2/1
  Rate Transition1/1 -> Decoupling1/3(wme)
  Circle Limitation/1(dq*) -> [UDQ], Rev_Park 2/1(dq)
  Demux/1 -> PI_curr2/1(id*)
  PI_curr2/1(Vdq*) -> Decoupling1/1(udq*)
  Decoupling1/1(udq**) -> Circle Limitation/1(dq)
  Demux/2 -> Gain/1
  Gain/1 -> PI_curr2/2(iq*)

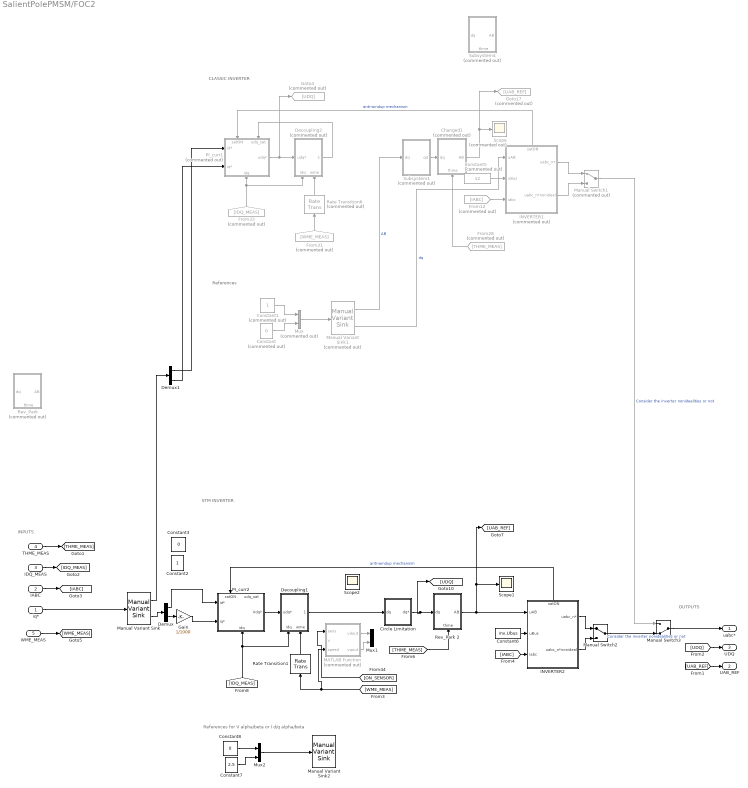
== system SalientPolePMSM/FOC2 ==
  note: References for V alpha/beta or I d/q alpha/beta
  note: OUTPUTS
  note: STM INVERTER
  note: INPUTS
  note: CLASSIC INVERTER
  note: References
  iq* : Inport
  IABC : Inport  Port=2
  IDQ_MEAS : Inport  Port=3
  THME_MEAS : Inport  Port=4
  WME_MEAS : Inport  Port=5
  Changed1 : Subsystem  Commented=on
      settings: PortSchema="{\"entries\":[{\"content\":{\"sides\":[{\"content\":{\"connectorIds\":[\"In1\"]},\"type\":\"ConnectorPlacement.EquallySpacedRectSide\",\"uuid\":\"ea71606c-027e-481e-aba4-13f62585a677\"},{\"content\":{\"connectorIds\":[\"Out1\"],\"side\":\"RIGHT\"},\"type\":\"ConnectorPlacement.EquallySpacedRectSide\",\"uuid\":\"049929a5-aa1b-4856-95c9-17d9e38685d8\"},{\"content\":{\"connectorIds\":[],\"side\":\"TOP\"},\"type\":\"ConnectorPlacement.EquallySpacedRectSide\",\"uuid\":\"6c7bede6-8f52-43d3-8925-2a8f1f9ce837\"},{\"content\":{\"connectorIds\":[\"In2\"],\"side\":\"BOTTOM\"},\"type\":\"ConnectorPlacement.EquallySpacedRectSide\",\"uuid\":\"34422c14-5aba-4255-be55-6ec9502f5391\"},{\"content\":{\"connectorIds\":[],\"side\":\"HIDDEN\"},\"type\":\"ConnectorPlacement.EquallySpacedRectSide\",\"uuid\":\"23931446-a8a1-432e-a504-22fe56898a45\"}]},\"type\":\"ConnectorPlacement.EquallySpacedConnector\",\"uuid\":\"f447a990-15af-42ca-9219-73ae62b099f5\"}],\"packageUris\":[\"http://schema.mathworks.com/mf0/Connector/R2020b\"],\"version\":\"1.0\"}"
  Circle Limitation : Subsystem
  Constant : Constant  Commented=on  Value=0  SampleTime=inv.Ts
  Constant1 : Constant  Commented=on  SampleTime=inv.Ts
  Constant2 : Constant  SampleTime=-1
  Constant3 : Constant  Value=0  SampleTime=-1
  Constant5 : Constant  Commented=on  Value=12
  Constant6 : Constant  Value=inv.Ubus
  Constant7 : Constant  Value=2.5  SampleTime=-1
  Constant8 : Constant  Value=0  SampleTime=-1
  Decoupling1 : Subsystem
      settings: PortSchema="{\"entries\":[{\"content\":{\"sides\":[{\"content\":{\"connectorIds\":[\"In1\"]},\"type\":\"ConnectorPlacement.EquallySpacedRectSide\",\"uuid\":\"366d4760-99ea-4839-93ce-cd028ffff2ed\"},{\"content\":{\"connectorIds\":[\"Out1\"],\"side\":\"RIGHT\"},\"type\":\"ConnectorPlacement.EquallySpacedRectSide\",\"uuid\":\"ffb80cd0-5569-4ccd-9b8e-dc37fbe2d6f7\"},{\"content\":{\"connectorIds\":[],\"side\":\"TOP\"},\"type\":\"ConnectorPlacement.EquallySpacedRectSide\",\"uuid\":\"2e02478e-0c74-4c41-9c3e-8c0e6bb6923b\"},{\"content\":{\"connectorIds\":[\"In2\",\"In3\"],\"side\":\"BOTTOM\"},\"type\":\"ConnectorPlacement.EquallySpacedRectSide\",\"uuid\":\"0c356034-c9d0-432b-942d-38470146113e\"}]},\"type\":\"ConnectorPlacement.EquallySpacedConnector\",\"uuid\":\"999d36d2-be3d-4c0f-9dc8-4c30e8aa3320\"}],\"packageUris\":[\"http://schema.mathworks.com/mf0/Connector/19700101\"],\"version\":\"1.0\"}"
  Decoupling2 : Subsystem  Commented=on
      settings: PortSchema="{\"entries\":[{\"content\":{\"sides\":[{\"content\":{\"connectorIds\":[\"In1\"]},\"type\":\"ConnectorPlacement.EquallySpacedRectSide\",\"uuid\":\"366d4760-99ea-4839-93ce-cd028ffff2ed\"},{\"content\":{\"connectorIds\":[\"Out1\"],\"side\":\"RIGHT\"},\"type\":\"ConnectorPlacement.EquallySpacedRectSide\",\"uuid\":\"ffb80cd0-5569-4ccd-9b8e-dc37fbe2d6f7\"},{\"content\":{\"connectorIds\":[],\"side\":\"TOP\"},\"type\":\"ConnectorPlacement.EquallySpacedRectSide\",\"uuid\":\"2e02478e-0c74-4c41-9c3e-8c0e6bb6923b\"},{\"content\":{\"connectorIds\":[\"In2\",\"In3\"],\"side\":\"BOTTOM\"},\"type\":\"ConnectorPlacement.EquallySpacedRectSide\",\"uuid\":\"0c356034-c9d0-432b-942d-38470146113e\"}]},\"type\":\"ConnectorPlacement.EquallySpacedConnector\",\"uuid\":\"999d36d2-be3d-4c0f-9dc8-4c30e8aa3320\"}],\"packageUris\":[\"http://schema.mathworks.com/mf0/Connector/19700101\"],\"version\":\"1.0\"}"
  Demux : Demux  Outputs=2
  Demux1 : Demux  Outputs=2
  From12 : From  Commented=on  GotoTag=IABC
  From28 : From  Commented=on  GotoTag=THME_MEAS
  From31 : From  Commented=on  GotoTag=WME_MEAS
  From33 : From  Commented=on  GotoTag=IDQ_MEAS
  Gain : Gain  Gain=1/1000
  Goto17 : Goto  Commented=on  GotoTag=UAB_REF
  Goto4 : Goto  Commented=on  GotoTag=UDQ
  INVERTER1 : Subsystem  Commented=on
      settings: PortSchema="{\"entries\":[{\"content\":{\"sides\":[{\"content\":{\"connectorIds\":[\"In1\",\"In2\",\"In3\"]},\"type\":\"ConnectorPlacement.EquallySpacedRectSide\",\"uuid\":\"79c77d12-022f-42ce-98d0-f3ead9d04a95\"},{\"content\":{\"connectorIds\":[\"Out1\",\"Out2\"],\"side\":\"RIGHT\"},\"type\":\"ConnectorPlacement.EquallySpacedRectSide\",\"uuid\":\"afd498dc-a72a-45ee-96a4-44488bf591ce\"},{\"content\":{\"connectorIds\":[\"Out3\"],\"side\":\"TOP\"},\"type\":\"ConnectorPlacement.EquallySpacedRectSide\",\"uuid\":\"f8f8ad46-d0da-4286-941c-855cc15ed51d\"}]},\"type\":\"ConnectorPlacement.EquallySpacedConnector\",\"uuid\":\"436ef73d-4718-409e-82fb-57ff2ccd93cf\"}],\"packageUris\":[\"http://schema.mathworks.com/mf0/Connector/R2020b\"],\"version\":\"1.0\"}"
  INVERTER2 : Subsystem
      settings: PortSchema="{\"entries\":[{\"content\":{\"sides\":[{\"content\":{\"connectorIds\":[\"In1\",\"In2\",\"In3\"]},\"type\":\"ConnectorPlacement.EquallySpacedRectSide\",\"uuid\":\"79c77d12-022f-42ce-98d0-f3ead9d04a95\"},{\"content\":{\"connectorIds\":[\"Out1\",\"Out2\"],\"side\":\"RIGHT\"},\"type\":\"ConnectorPlacement.EquallySpacedRectSide\",\"uuid\":\"afd498dc-a72a-45ee-96a4-44488bf591ce\"},{\"content\":{\"connectorIds\":[\"Out3\"],\"side\":\"TOP\"},\"type\":\"ConnectorPlacement.EquallySpacedRectSide\",\"uuid\":\"f8f8ad46-d0da-4286-941c-855cc15ed51d\"}]},\"type\":\"ConnectorPlacement.EquallySpacedConnector\",\"uuid\":\"436ef73d-4718-409e-82fb-57ff2ccd93cf\"}],\"packageUris\":[\"http://schema.mathworks.com/mf0/Connector/R2020b\"],\"version\":\"1.0\"}"
  MATLAB Function : MATLAB Function  Commented=on  TreatAsAtomicUnit=on  SystemSampleTime=inv.Ts
  Manual Variant Sink : simulink/Signal Routing/Manual Variant Sink  NumChoices=2  LabelModeActiveChoice=V_2
  Manual Variant Sink1 : simulink/Signal Routing/Manual Variant Sink  Commented=on  NumChoices=2  LabelModeActiveChoice=V_2
  Manual Variant Sink2 : simulink/Signal Routing/Manual Variant Sink  NumChoices=2  LabelModeActiveChoice=V_1
  Manual Switch1 : ManualSwitch  Commented=on
  Manual Switch2 : ManualSwitch
  Manual Switch3 : ManualSwitch  CurrentSetting=0
  Mux : Mux  Commented=on  Inputs=2
  Mux1 : Mux  Inputs=2
  Mux2 : Mux  Inputs=2
  PI_curr1 : Subsystem  Commented=on
      settings: PortSchema="{\"entries\":[{\"content\":{\"sides\":[{\"content\":{\"connectorIds\":[\"In1\",\"In2\"]},\"type\":\"ConnectorPlacement.EquallySpacedRectSide\",\"uuid\":\"366d4760-99ea-4839-93ce-cd028ffff2ed\"},{\"content\":{\"connectorIds\":[\"Out1\"],\"side\":\"RIGHT\"},\"type\":\"ConnectorPlacement.EquallySpacedRectSide\",\"uuid\":\"ffb80cd0-5569-4ccd-9b8e-dc37fbe2d6f7\"},{\"content\":{\"connectorIds\":[\"In3\",\"In4\"],\"side\":\"TOP\"},\"type\":\"ConnectorPlacement.EquallySpacedRectSide\",\"uuid\":\"2e02478e-0c74-4c41-9c3e-8c0e6bb6923b\"},{\"content\":{\"connectorIds\":[\"In5\"],\"side\":\"BOTTOM\"},\"type\":\"ConnectorPlacement.EquallySpacedRectSide\",\"uuid\":\"f2f25d95-a140-4291-ad57-573bdd6b43a2\"}]},\"type\":\"ConnectorPlacement.EquallySpacedConnector\",\"uuid\":\"999d36d2-be3d-4c0f-9dc8-4c30e8aa3320\"}],\"packageUris\":[\"http://schema.mathworks.com/mf0/Connector/R2020b\"],\"version\":\"1.0\"}"
  PI_curr2 : Subsystem
      settings: PortSchema="{\"entries\":[{\"content\":{\"sides\":[{\"content\":{\"connectorIds\":[\"In1\",\"In2\"]},\"type\":\"ConnectorPlacement.EquallySpacedRectSide\",\"uuid\":\"366d4760-99ea-4839-93ce-cd028ffff2ed\"},{\"content\":{\"connectorIds\":[\"Out1\"],\"side\":\"RIGHT\"},\"type\":\"ConnectorPlacement.EquallySpacedRectSide\",\"uuid\":\"ffb80cd0-5569-4ccd-9b8e-dc37fbe2d6f7\"},{\"content\":{\"connectorIds\":[\"In3\",\"In4\"],\"side\":\"TOP\"},\"type\":\"ConnectorPlacement.EquallySpacedRectSide\",\"uuid\":\"2e02478e-0c74-4c41-9c3e-8c0e6bb6923b\"},{\"content\":{\"connectorIds\":[\"In5\"],\"side\":\"BOTTOM\"},\"type\":\"ConnectorPlacement.EquallySpacedRectSide\",\"uuid\":\"f2f25d95-a140-4291-ad57-573bdd6b43a2\"}]},\"type\":\"ConnectorPlacement.EquallySpacedConnector\",\"uuid\":\"999d36d2-be3d-4c0f-9dc8-4c30e8aa3320\"}],\"packageUris\":[\"http://schema.mathworks.com/mf0/Connector/R2020b\"],\"version\":\"1.0\"}"
  Rate Transition1 : RateTransition  OutPortSampleTime=PI.cur.Ts
  Rate Transition6 : RateTransition  Commented=on  OutPortSampleTime=PI.cur.Ts
  Rev_Park : Subsystem  Commented=on
      settings: PortSchema="{\"entries\":[{\"content\":{\"sides\":[{\"content\":{\"connectorIds\":[\"In1\"]},\"type\":\"ConnectorPlacement.EquallySpacedRectSide\",\"uuid\":\"ea71606c-027e-481e-aba4-13f62585a677\"},{\"content\":{\"connectorIds\":[\"Out1\"],\"side\":\"RIGHT\"},\"type\":\"ConnectorPlacement.EquallySpacedRectSide\",\"uuid\":\"049929a5-aa1b-4856-95c9-17d9e38685d8\"},{\"content\":{\"connectorIds\":[],\"side\":\"TOP\"},\"type\":\"ConnectorPlacement.EquallySpacedRectSide\",\"uuid\":\"6c7bede6-8f52-43d3-8925-2a8f1f9ce837\"},{\"content\":{\"connectorIds\":[\"In2\"],\"side\":\"BOTTOM\"},\"type\":\"ConnectorPlacement.EquallySpacedRectSide\",\"uuid\":\"34422c14-5aba-4255-be55-6ec9502f5391\"},{\"content\":{\"connectorIds\":[],\"side\":\"HIDDEN\"},\"type\":\"ConnectorPlacement.EquallySpacedRectSide\",\"uuid\":\"23931446-a8a1-432e-a504-22fe56898a45\"}]},\"type\":\"ConnectorPlacement.EquallySpacedConnector\",\"uuid\":\"f447a990-15af-42ca-9219-73ae62b099f5\"}],\"packageUris\":[\"http://schema.mathworks.com/mf0/Connector/R2020b\"],\"version\":\"1.0\"}"
  Rev_Park 2 : Subsystem
      settings: PortSchema="{\"entries\":[{\"content\":{\"sides\":[{\"content\":{\"connectorIds\":[\"In1\"]},\"type\":\"ConnectorPlacement.EquallySpacedRectSide\",\"uuid\":\"ea71606c-027e-481e-aba4-13f62585a677\"},{\"content\":{\"connectorIds\":[\"Out1\"],\"side\":\"RIGHT\"},\"type\":\"ConnectorPlacement.EquallySpacedRectSide\",\"uuid\":\"049929a5-aa1b-4856-95c9-17d9e38685d8\"},{\"content\":{\"connectorIds\":[],\"side\":\"TOP\"},\"type\":\"ConnectorPlacement.EquallySpacedRectSide\",\"uuid\":\"6c7bede6-8f52-43d3-8925-2a8f1f9ce837\"},{\"content\":{\"connectorIds\":[\"In2\"],\"side\":\"BOTTOM\"},\"type\":\"ConnectorPlacement.EquallySpacedRectSide\",\"uuid\":\"34422c14-5aba-4255-be55-6ec9502f5391\"},{\"content\":{\"connectorIds\":[],\"side\":\"HIDDEN\"},\"type\":\"ConnectorPlacement.EquallySpacedRectSide\",\"uuid\":\"23931446-a8a1-432e-a504-22fe56898a45\"}]},\"type\":\"ConnectorPlacement.EquallySpacedConnector\",\"uuid\":\"f447a990-15af-42ca-9219-73ae62b099f5\"}],\"packageUris\":[\"http://schema.mathworks.com/mf0/Connector/R2020b\"],\"version\":\"1.0\"}"
  Scope : Scope  Commented=on
  Scope1 : Scope
  Scope2 : Scope
  Subsystem1 : Subsystem  Commented=on
  Subsystem4 : Subsystem  Commented=on
      settings: PortSchema="{\"entries\":[{\"content\":{\"sides\":[{\"content\":{\"connectorIds\":[\"In1\"]},\"type\":\"ConnectorPlacement.EquallySpacedRectSide\",\"uuid\":\"ea71606c-027e-481e-aba4-13f62585a677\"},{\"content\":{\"connectorIds\":[\"Out1\"],\"side\":\"RIGHT\"},\"type\":\"ConnectorPlacement.EquallySpacedRectSide\",\"uuid\":\"049929a5-aa1b-4856-95c9-17d9e38685d8\"},{\"content\":{\"connectorIds\":[],\"side\":\"TOP\"},\"type\":\"ConnectorPlacement.EquallySpacedRectSide\",\"uuid\":\"6c7bede6-8f52-43d3-8925-2a8f1f9ce837\"},{\"content\":{\"connectorIds\":[\"In2\"],\"side\":\"BOTTOM\"},\"type\":\"ConnectorPlacement.EquallySpacedRectSide\",\"uuid\":\"34422c14-5aba-4255-be55-6ec9502f5391\"},{\"content\":{\"connectorIds\":[],\"side\":\"HIDDEN\"},\"type\":\"ConnectorPlacement.EquallySpacedRectSide\",\"uuid\":\"23931446-a8a1-432e-a504-22fe56898a45\"}]},\"type\":\"ConnectorPlacement.EquallySpacedConnector\",\"uuid\":\"f447a990-15af-42ca-9219-73ae62b099f5\"}],\"packageUris\":[\"http://schema.mathworks.com/mf0/Connector/R2020b\"],\"version\":\"1.0\"}"
  uabc* : Outport
  UAB_REF : Outport  Port=2
  UDQ : Outport  Port=3
  wires:
  Constant6/1 -> INVERTER2/2(uBus)
  INVERTER2/3(satON) -> PI_curr2/3(satON)  "anti-windup mechanism"
  INVERTER2/1(uabc_n*) -> Manual Switch2/1
  INVERTER2/2(uabc_n*nonideal) -> Manual Switch2/2
  [IABC] -> INVERTER2/3(iabc)
  [IDQ_MEAS] -> Decoupling1/2(idq), PI_curr2/5(idq)
  Constant/1 -> Mux/2
  Constant1/1 -> Mux/1
  Demux1/1 -> PI_curr1/1(id*)
  [UDQ] -> UDQ/1
  THME_MEAS/1 -> [THME_MEAS]
  IDQ_MEAS/1 -> [IDQ_MEAS]
  IABC/1 -> [IABC]
  [UAB_REF] -> UAB_REF/1
  Decoupling2/1(udq**) -> PI_curr1/4(udq_sat)
  Rate Transition6/1 -> Decoupling2/3(wme)
  Constant5/1 -> INVERTER1/2(uBus)
  INVERTER1/1(uabc_n*) -> Manual Switch1/1
  From28/1 -> Changed1/2(thme)
  INVERTER1/2(uabc_n*nonideal) -> Manual Switch1/2
  INVERTER1/3(satON) -> PI_curr1/3(satON)  "anti-windup mechanism"
  Changed1/1(AB) -> Scope/1, Goto17/1
  From31/1 -> Rate Transition6/1
  From33/1 -> Decoupling2/2(idq), PI_curr1/5(idq)
  From12/1 -> INVERTER1/3(iabc)
  PI_curr1/1(udq*) -> Decoupling2/1(udq*), Goto4/1
  Subsystem1/1(qd) -> Changed1/1(dq)
  [WME_MEAS] -> MATLAB Function/3(speed), Rate Transition1/1
  Manual Switch3/1 -> uabc*/1
  Manual Switch2/1 -> Manual Switch3/2  "Consider the inverter nonidealities or not"
  Manual Switch1/1 -> Manual Switch3/1  "Consider the inverter nonidealities or not"
  iq*/1 -> Manual Variant Sink/1
  Mux/1 -> Manual Variant Sink1/1
  Manual Variant Sink1/1 -> Subsystem1/1(dq)  "AB"
  Manual Variant Sink1/2 -> INVERTER1/1(uAB)  "dq"
  Mux2/1 -> Manual Variant Sink2/1
  Rev_Park 2/1(AB) -> INVERTER2/1(uAB), [UAB_REF], Scope1/1
  Manual Variant Sink/2 -> Demux/1
  Manual Variant Sink/1 -> Demux1/1
  Demux1/2 -> PI_curr1/2(iq*)
  WME_MEAS/1 -> [WME_MEAS]
  [THME_MEAS] -> Rev_Park 2/2(thme)
  [ON_SENSOR] -> MATLAB Function/1(sens)
  MATLAB Function/2(vqout) -> Mux1/2
  MATLAB Function/1(vdout) -> Mux1/1
  Constant7/1 -> Mux2/2
  Constant8/1 -> Mux2/1
  Rate Transition1/1 -> Decoupling1/3(wme)
  Circle Limitation/1(dq*) -> [UDQ], Rev_Park 2/1(dq)
  Demux/1 -> PI_curr2/1(id*)
  PI_curr2/1(Vdq*) -> Decoupling1/1(udq*)
  Decoupling1/1(udq**) -> Circle Limitation/1(dq)
  Demux/2 -> Gain/1
  Gain/1 -> PI_curr2/2(iq*)
